simulink model "Exercise111"  (R2017a)
settings: Solver=VariableStepAuto  StartTime=0.0  StopTime=10.0  RelTol=1e-3
undefined symbols (not defined in the file): Den, Fin_Val, Num, Step_Time
settings Model: Creator=JakobLab  LastModifiedBy=JakobLab

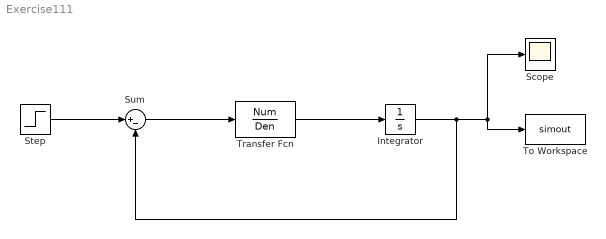
== system Exercise111 ==
  Integrator : Integrator
  Scope : Scope
  Step : Step  Time=Step_Time  After=Fin_Val  SampleTime=0
  Sum : Sum  Inputs=|+-
  To Workspace : ToWorkspace  VariableName=simout  SaveFormat=Structure With Time  SampleTime=-1
  Transfer Fcn : TransferFcn  Numerator=Num  Denominator=Den
  wires:
  Step/1 -> Sum/1
  Sum/1 -> Transfer Fcn/1
  Transfer Fcn/1 -> Integrator/1
  Integrator/1 -> Sum/2, To Workspace/1, Scope/1
